simulink model "LikestromsmotorSimulinkVariables"  (R2023a)
settings: Solver=VariableStepAuto  StartTime=0.0  StopTime=10  RelTol=1e-3
libraries: slpidlib x1
settings Model: Creator=augus  LastModifiedBy=augus

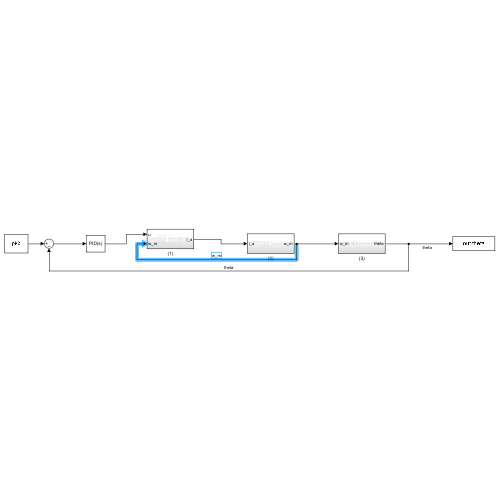
[thumbnail: Simulink's stored preview of the top-level diagram]
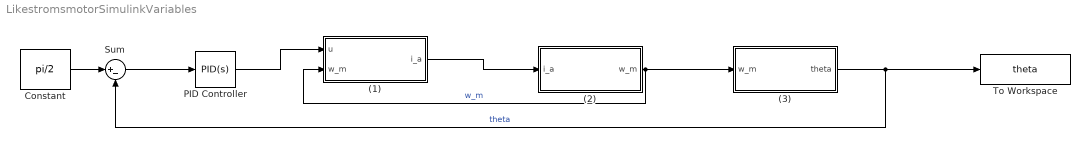
== system LikestromsmotorSimulinkVariables ==
  (1) : Subsystem
  (2) : Subsystem
  (3) : Subsystem
  Constant : Constant  Value=pi/2
  PID Controller : slpidlib/PID Controller  Controller=PID  Form=Ideal  TimeDomain=Continuous-time  UseExternalTs=off  SampleTime=-1  IntegratorMethod=Forward Euler  FilterMethod=Forward Euler  ControllerParametersSource=internal  P=5.97  I=0.3  UseKiTs=off  D=0.075  N=1000  UseFilter=on  TunerSelectOption=Frequency Response Based  InitialConditionSource=internal  InitialConditionForIntegrator=0  InitialConditionForFilter=0  DifferentiatorICPrevScaledInput=0  ExternalReset=none  TrackingMode=off  Kt=1  LimitOutput=off  SatLimitsSource=internal  UpperSaturationLimit=inf  LowerSaturationLimit=-inf  LinearizeAsGain=on  AntiWindupMode=none  Kb=1  LimitIntegrator=off  UpperIntegratorSaturationLimit=inf  LowerIntegratorSaturationLimit=-inf  POutMin=[]  POutMax=[]  IOutMin=[]  IOutMax=[]  DOutMin=[]  DOutMax=[]  NOutMin=[]  NOutMax=[]  SumOutMin=[]  SumOutMax=[]  SaturationOutMin=[]  SaturationOutMax=[]  PParamMin=[]  PParamMax=[]  IParamMin=[]  IParamMax=[]  DParamMin=[]  DParamMax=[]  NParamMin=[]  NParamMax=[]  KbParamMin=[]  KbParamMax=[]  KtParamMin=[]  KtParamMax=[]  KbOutMin=[]  KbOutMax=[]  KtOutMin=[]  KtOutMax=[]  IntegratorOutMin=[]  IntegratorOutMax=[]  FilterOutMin=[]  FilterOutMax=[]  SumI1OutMin=[]  SumI1OutMax=[]  SumI2OutMin=[]  SumI2OutMax=[]  SumI3OutMin=[]  SumI3OutMax=[]  SumI4OutMin=[]  SumI4OutMax=[]  SumDOutMin=[]  SumDOutMax=[]  DifferentiatorOutMin=[]  DifferentiatorOutMax=[]  FilterDiffOutCoefMin=[]  FilterDiffOutCoefMax=[]  ReciprocalOutMin=[]  ReciprocalOutMax=[]  SumDenOutMin=[]  SumDenOutMax=[]  SumNumOutMin=[]  SumNumOutMax=[]  DivideOutMin=[]  DivideOutMax=[]  UdiffTsProdOutMin=[]  UdiffTsProdOutMax=[]  NTsProdOutMin=[]  NTsProdOutMax=[]  UintegralTsProdOutMin=[]  UintegralTsProdOutMax=[]  UngainTsProdOutMin=[]  UngainTsProdOutMax=[]  ClampingZeroOutDataTypeStr=Inherit: Inherit via back propagation  ClampingZeroOutMin=[]  ClampingZeroOutMax=[]  FilterDenConstantOutDataTypeStr=Inherit: Inherit via back propagation  FilterDenConstantOutMin=[]  FilterDenConstantOutMax=[]  PCopyOutDataTypeStr=Inherit: Inherit via back propagation  PCopyOutMin=[]  PCopyOutMax=[]  NCopyOutDataTypeStr=Inherit: Inherit via back propagation  NCopyOutMin=[]  NCopyOutMax=[]  IntegratorContinuousStateAttributes=''  IntegratorStateMustResolveToSignalObject=off  IntegratorRTWStateStorageClass=Auto  FilterContinuousStateAttributes=''  FilterStateMustResolveToSignalObject=off  FilterRTWStateStorageClass=Auto  ParallelPVariant=Passthrough  IdealPVariant=InternalParameters  IVariant=InternalParameters  DVariant=InternalParameters  IntegratorVariant=Continuous  SatVariant=Disabled  AWVariant=Passthrough  PCopyVariant=Disabled  TRVariant=Disabled  FdbkBlocksVariant=Forward  IdealPFdbkVariant=Disabled  SatFdbkVariant=Disabled  DerivativeFilterVariant=ContFilter  NVariant=InternalParameters  NCopyVariant=Disabled  FilterICVariant=InternalICsFilter  IntegratorICVariant=InternalICs  ExternalResetVariant=Disabled  TRSumVariant=Passthrough  SumFdbkVariant=Disabled  SumVariant=Sum_PID  TsampFilterVariant=InternalTs  TsampNgainVariant=Passthrough  TsampIntegralVariant=Disabled_SignalSpec  ExternalSaturationOutDataTypeStr=Inherit: Same as second input
  Sum : Sum  Inputs=|+-
  To Workspace : ToWorkspace  VariableName=theta  SaveFormat=Timeseries  SampleTime=-1
  wires:
  (2)/1(w_m) -> (1)/2(w_m), (3)/1(w_m)  "w_m"
  PID Controller/1 -> (1)/1(u)
  Constant/1 -> Sum/1
  Sum/1 -> PID Controller/1
  (3)/1(theta) -> Sum/2, To Workspace/1  "theta"
  (1)/1(i_a) -> (2)/1(i_a)

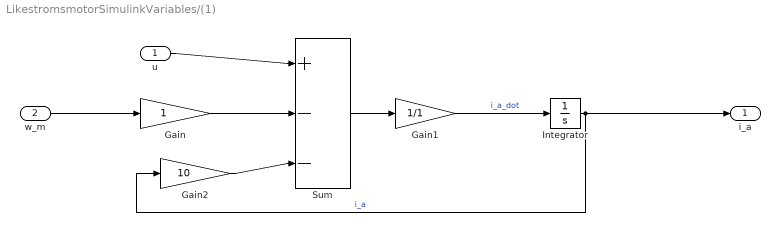
== system LikestromsmotorSimulinkVariables/(1) ==
  u : Inport
  w_m : Inport  Port=2
  Gain : Gain
  Gain1 : Gain  Gain=1/1
  Gain2 : Gain  Gain=10
  Integrator : Integrator
  Sum : Sum  Inputs=+|-|-
  i_a : Outport
  wires:
  u/1 -> Sum/1
  Gain/1 -> Sum/2
  w_m/1 -> Gain/1
  Sum/1 -> Gain1/1
  Gain1/1 -> Integrator/1  "i_a_dot"
  Gain2/1 -> Sum/3
  Integrator/1 -> Gain2/1, i_a/1  "i_a"

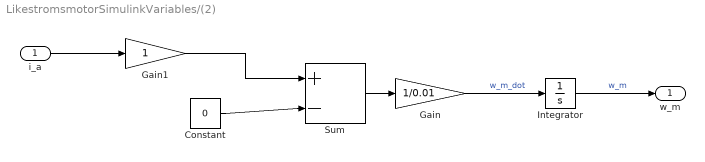
== system LikestromsmotorSimulinkVariables/(2) ==
  i_a : Inport
  Constant : Constant  Value=0
  Gain : Gain  Gain=1/0.01
  Gain1 : Gain
  Integrator : Integrator
  Sum : Sum  Inputs=+|-
  w_m : Outport
  wires:
  Sum/1 -> Gain/1
  Integrator/1 -> w_m/1  "w_m"
  Gain/1 -> Integrator/1  "w_m_dot"
  Constant/1 -> Sum/2
  Gain1/1 -> Sum/1
  i_a/1 -> Gain1/1

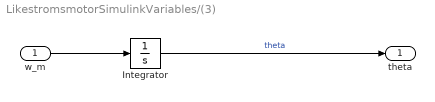
== system LikestromsmotorSimulinkVariables/(3) ==
  w_m : Inport
  Integrator : Integrator
  theta : Outport
  wires:
  w_m/1 -> Integrator/1
  Integrator/1 -> theta/1  "theta"
